simulink model "tqdtqr_rebuild_V3"  (R2021b)
settings: Solver=VariableStepAuto  StartTime=0.0  StopTime=10.0  RelTol=1e-3
undefined symbols (not defined in the file): ATQD_AfterTqMinGain_X_Deg, ATQD_APSCreepBaseTqD_X_kph, ATQD_APSCreepBaseTqD_Y_Deg, ATQD_APSCreepBaseTqR_X_kph, ATQD_APSCreepBaseTqR_Y_Deg, ATQD_APSCreepIterm_X_kph, ATQD_APSCreepIterm_Y_kph, ATQD_APSCreepPterm_X_kph, ATQD_APSCreepPterm_Y_kph, ATQD_APSDecReq_X_kph, ATQD_APSDecReq_Y_mps2, ATQD_APSDecReqCMD_X_kph, ATQD_APSDecReqTs_X_pct, ATQD_APSDecTimeGain_X_Deg, ATQD_APSDecTimeGain_Y_s, ATQD_APSReqLowSpd_X_Deg, ATQD_AutoHoldReleaseBPS_X_Deg, ATQD_AWDLoadTrqnsGain_X_kg, ATQD_AWDLoadTrqnsGain_Y_pct, ATQD_BOSEnBPSPosn_X_kph, ATQD_BOSMap_X_rpm, ATQD_BOSMap_Y_pct, ATQD_CreepBaseTqD_X_kph, ATQD_CreepBaseTqD_Y_Deg, ATQD_CreepBaseTqR_X_kph, ATQD_CreepBaseTqR_Y_Deg, ATQD_CreepBPSDisPosn_X_Deg, ATQD_CreepBPSDisPosnR_X_Deg, ATQD_CreepBPSEnPosn_X_Deg, ATQD_CreepBPSEnPosnR_X_Deg, ATQD_CreepDeltaTq_X_kph, ATQD_CreepIterm_X_kph, ATQD_CreepIterm_Y_kph, ATQD_CreepItermMaxLimit_X_pct, ATQD_CreepPreloadTime_X_kph, ATQD_CreepPreloadTq_X_kph, ATQD_CreepPreloadTq_Y_s, ATQD_CreepProtTq_X_Deg, ATQD_CreepPterm_X_kph, ATQD_CreepPterm_Y_kph, ATQD_CreepRrTqSpRat_X_rpm, ATQD_CreepRrTqSpRat_Y_Nm, ATQD_CreepTargetSpdD_X_pct, ATQD_CreepTargetSpdR_X_pct, ATQD_CreepUpLimitTq_X_rpm, ATQD_DecIneOPDHoldEnDelay_X_Deg, ATQD_DecIneOPDHoldEnDelay_Y_bar, ATQD_ECOTqMapD_X_rpm, ATQD_ECOTqMapD_Y_pct, ATQD_EMTqMapD_X_rpm, ATQD_EMTqMapD_Y_pct, ATQD_EOPDTqMapDCon_X_rpm, ATQD_EOPDTqMapDCon_Y_Deg, ATQD_EstInitVehWeight_X_c, ATQD_FAfterTqCMDGain_X_rpm, ATQD_FAfterTqCMDGain_Y_pct, ATQD_ForceLowSpd_X_Deg, ATQD_ForcePLimitSpd_X_Deg, ATQD_FrLossMAPLowV_X_rpm, ATQD_FrLossMAPLowV_Y_Nm ... (+949)
libraries: simulink x235, hcu_lib x208, tqr x63, tqd x6
(part 29 of 37)

== system tqdtqr_rebuild_V3/Input_Convert/Signal function/VehWeightEst/Calaulation/Rear Wheel Torque ==
  VINP_RrEDURealTMTq_Nm : Inport
  VTQD_VehWeightEstEn_flg : Inport  Port=2
  VTQD_VehWeightEstDis_flg : Inport  Port=3
  VTQD_VehWeightEstEnd_flg : Inport  Port=4
  task_time_s : Inport  Port=5
  AND : Logic  AllPortsSameDT=off  OutDataTypeStr=boolean
  AND1 : Logic  AllPortsSameDT=off  OutDataTypeStr=boolean
  AND2 : Logic  AllPortsSameDT=off  OutDataTypeStr=boolean
  Abs : Abs
  Add : Sum
  Add1 : Sum
  Add2 : Sum  Inputs=+-
  Constant1 : Constant  Value=ZERO_FLOAT
  Constant2 : Constant  Value=KTQD_VehWeighEstTime_s
  Constant3 : Constant  Value=ZERO_FLOAT
  Constant4 : Constant  Value=KTQD_VehWeighEstTimeTune_cnt
  Constant5 : Constant  Value=ZERO_FLOAT
  Constant6 : Constant  Value=KTQD_EstRrWhlTqDev_Nm
  Data Type Conversion : DataTypeConversion  OutDataTypeStr=uint8
  Delay : Delay  DelayLength=1  InitialCondition=boolean(0)
      settings: AttributesFormatString=%<InitialCondition>
  Delay1 : Delay  DelayLength=1  InitialCondition=single(0.0)
      settings: AttributesFormatString=%<InitialCondition>
  Delay2 : Delay  DelayLength=1
  Delay3 : Delay  DelayLength=1  InitialCondition=boolean(0)
      settings: AttributesFormatString=%<InitialCondition>
  Delay4 : Delay  DelayLength=1  InitialCondition=single(0.0)
      settings: AttributesFormatString=%<InitialCondition>
  Detect Decrease : simulink/Logic and Bit Operations/Detect Decrease  vinit=boolean(0)  OutDataTypeStr=boolean
  Detect Increase : simulink/Logic and Bit Operations/Detect Increase  vinit=boolean(0)  OutDataTypeStr=boolean
  Divide : Product  Inputs=*/
  Divide1 : Product  Inputs=*/
  Min : MinMax  Inputs=2
  NOT : Logic  Operator=NOT  AllPortsSameDT=off  OutDataTypeStr=boolean
  NOT1 : Logic  Operator=NOT  AllPortsSameDT=off  OutDataTypeStr=boolean
  Relational Operator : RelationalOperator  Operator=<=  OutDataTypeStr=boolean  RndMeth=Simplest
  Switch : Switch  Criteria=u2 ~= 0
  Switch1 : Switch  Criteria=u2 ~= 0
  Switch2 : Switch  Criteria=u2 > Threshold
  Switch3 : Switch  Criteria=u2 ~= 0
      settings: AttributesFormatString=%<Criteria>
  Terminator : Terminator
  VTQD_EstRrRealTqAvg_Nm : Outport
  VTQD_EstRrRealTqCheckPass_flg : Outport  Port=2
  wires:
  [VTQD_EstRrRealTqAvg_Nm] -> VTQD_EstRrRealTqAvg_Nm/1
  [VTQD_EstRrRealTqCheckPass_flg] -> VTQD_EstRrRealTqCheckPass_flg/1
  Constant4/1 -> Add1/2
  [VINP_RrEDURealTMTq_Nm] -> Min/1
  Delay1/1 -> Add/2
  Constant3/1 -> Switch2/1
  [VTQD_VehWeightEstEn_flg] -> AND/1
  Divide1/1 -> [VTQD_EstRrRealTqAvg_Nm]  "VTQD_EstRrRealTqAvg_Nm"
  Switch/1 -> Add/1
  [VTQD_EstRrRealTqSum_Nm] -> Divide1/1
  [VTQD_VehWeightEstEn_flg] -> Detect Decrease/1
  AND/1 -> Switch/2
  Constant1/1 -> Switch/3
  [VTQD_VehWeightEstEn_flg] -> Detect Increase/1
  Relational Operator/1 -> AND1/2
  Add/1 -> Switch1/3
  Constant6/1 -> Relational Operator/2
  [VTQD_EstRrRealTqAvg_Nm] -> Add2/1
  [VINP_RrEDURealTMTq_Nm] -> Switch/1
  NOT/1 -> AND/2
  Constant5/1 -> Switch1/1
  Switch1/1 -> [VTQD_EstRrRealTqSum_Nm], Delay1/1  "VTQD_EstRrRealTqSum_Nm"
  Switch2/1 -> Delay4/1, [VTQD_EstRrRealTqMin_Nm]  "VTQD_EstRrRealTqMin_Nm"
  Constant2/1 -> Divide/1
  [VTQD_EstRrRealTqMin_Nm] -> Add2/2
  [VTQD_VehWeightEstDis_flg] -> Delay/1
  Delay2/1 -> Min/2
  [VTQD_EstRrRealTqMin_Nm] -> Delay2/1
  [task_time_s] -> Divide/2
  Detect Increase/1 -> Switch2/2
  Delay/1 -> NOT/1
  Abs/1 -> Relational Operator/1
  Add2/1 -> Abs/1
  [VTQD_VehWeightEstDis_flg] -> AND1/1
  AND1/1 -> [VTQD_EstRrRealTqCheckPass_flg]  "VTQD_EstRrRealTqCheckPass_flg"
  VINP_RrEDURealTMTq_Nm/1 -> [VINP_RrEDURealTMTq_Nm]
  VTQD_VehWeightEstEn_flg/1 -> [VTQD_VehWeightEstEn_flg]
  VTQD_VehWeightEstDis_flg/1 -> [VTQD_VehWeightEstDis_flg]
  VTQD_VehWeightEstEnd_flg/1 -> Terminator/1
  task_time_s/1 -> [task_time_s]
  Add1/1 -> Divide1/2  "VTQD_EstCycleCount_cnt"
  Divide/1 -> Data Type Conversion/1
  Data Type Conversion/1 -> Add1/1
  [VTQD_VehWeightEstEn_flg] -> AND2/1
  NOT1/1 -> AND2/2
  Delay3/1 -> NOT1/1
  [VTQD_VehWeightEstDis_flg] -> Delay3/1
  AND2/1 -> Switch3/2
  Min/1 -> Switch3/1
  Switch3/1 -> Switch2/3
  Delay4/1 -> Switch3/3
  Detect Decrease/1 -> Switch1/2

== system tqdtqr_rebuild_V3/Input_Convert/Signal function/VehWeightEst/Calaulation/Vehicle Weight ==
  VTQD_EstFrRealTqAvg_Nm : Inport
  VTQD_EstRrRealTqAvg_Nm : Inport  Port=2
  VTQD_EstLongAccAvg_Gps : Inport  Port=3
  VINP_VehSpeed_kph : Inport  Port=4
  Add : Sum  Inputs=+++
  Add1 : Sum
  Add2 : Sum
  Add3 : Sum
  Constant1 : Constant  Value=KTQD_RrTMTotalGearRatio_gain
  Constant10 : Constant  Value=KTQR_FrTMGearEff_c
  Constant11 : Constant  Value=KTQR_RrTMGearEff_c
  Constant12 : Constant  Value=MINUSONE_FLOAT
  Constant13 : Constant  Value=KTQD_GravityValue_mps2
  Constant2 : Constant  Value=KTQD_FrTMTotalGearRatio_gain
  Constant3 : Constant  Value=MINUSONE_FLOAT
  Constant4 : Constant  Value=MINUSONE_FLOAT
  Constant5 : Constant  Value=KTQD_FrTireRadius_m
  Constant6 : Constant  Value=KTQD_RrTireRadius_m
  Constant7 : Constant  Value=KTQD_EstRollCoeffA_c
  Constant8 : Constant  Value=KTQD_EstRollCoeffB_c
  Constant9 : Constant  Value=KTQD_EstRollCoeffC_c
  Divide : Product  Inputs=*/
  Divide1 : Product  Inputs=*/
  Divide2 : Product  Inputs=*/
  Product{,3..5} (4 alike) : Product
  Product1 : Product  Inputs=3
  Product2 : Product  Inputs=3
  Product6 : Product  Inputs=3
  Square : Math  Operator=square  SaturateOnIntegerOverflow=on
  VTQD_EstVehWeight_kg : Outport
  wires:
  [VINP_VehSpeed_kph] -> Square/1
  Divide/1 -> Add1/1  "VTQD_EstFrForce_N"
  Product2/1 -> Divide2/1  "VTQD_EstRrWhlTqAvg_Nm"
  [VINP_VehSpeed_kph] -> Product/2
  Constant6/1 -> Divide2/2
  Product1/1 -> Divide/1  "VTQD_EstFrWhlTqAvg_Nm"
  Constant2/1 -> Product1/2
  Constant1/1 -> Product2/2
  Add1/1 -> Product4/1
  Square/1 -> Product3/2
  [VTQD_EstRrRealTqAvg_Nm] -> Product2/1
  Constant3/1 -> Product1/3
  [VTQD_EstRollForce_N] -> Add2/2
  Constant9/1 -> Product3/1
  Constant7/1 -> Add/1
  [VTQD_EstFrRealTqAvg_Nm] -> Product1/1
  Constant10/1 -> Product4/2
  Add2/1 -> Product5/1
  Product4/1 -> Add3/1  "VTQD_EstFrActForce_N"
  Constant5/1 -> Divide/2
  Add/1 -> [VTQD_EstRollForce_N]  "VTQD_EstRollForce_N"
  Product/1 -> Add/2
  Constant4/1 -> Product2/3
  Add3/1 -> [VTQD_EstActTotalForce_N]  "VTQD_EstActTotalForce_N"
  Product5/1 -> Add3/2  "VTQD_EstRrActForce_N"
  Constant8/1 -> Product/1
  Divide2/1 -> Add2/1  "VTQD_EstRrForce_N"
  Constant11/1 -> Product5/2
  [VTQD_EstRollForce_N] -> Add1/2
  Product3/1 -> Add/3
  [VTQD_EstLongAccAvg_Gps] -> Product6/1
  Constant12/1 -> Product6/2
  Product6/1 -> Divide1/2
  [VTQD_EstActTotalForce_N] -> Divide1/1
  VTQD_EstFrRealTqAvg_Nm/1 -> [VTQD_EstFrRealTqAvg_Nm]
  VTQD_EstRrRealTqAvg_Nm/1 -> [VTQD_EstRrRealTqAvg_Nm]
  VTQD_EstLongAccAvg_Gps/1 -> [VTQD_EstLongAccAvg_Gps]
  VINP_VehSpeed_kph/1 -> [VINP_VehSpeed_kph]
  [VTQD_EstVehWeight_kg] -> VTQD_EstVehWeight_kg/1
  Constant13/1 -> Product6/3
  Divide1/1 -> [VTQD_EstVehWeight_kg]  "VTQD_EstVehWeight_kg"

== system tqdtqr_rebuild_V3/Input_Convert/Signal function/combo key/Combo Key Detection/DiagnosisOff Mode ==
  note: Check value key1~8 and diagnosis off mode on
  note: Detect combo key value from key1~8
  note: Exhibition Mode:
      | 1 = VINP_SWC2RegenDown_flg
      | 2 = VINP_SWC2RegenUp_flg
      | 3 = VINP_SWC2LScrollUpSta_flg
      | 4 = VINP_SWC2LScrollDownSta_flg
      | 5 = VINP_SWC2RScrollUpSta_flg
      | 6 = VINP_SWC2RScrollDownSta_flg
      | 7 = VINP_SWC2LScrollPressSta_flg
      | 8 = VINP_SWC2LADASSta_flg
  TASK_TIME_10_MS : Inport
  VSCP_ComboKeyEn_flg : Inport  Port=2
  VSCP_ComboKeyReset_flg : Inport  Port=3
  VSCP_ComboKey_enum : Inport  Port=4
  VSCP_ComboKeyEnter_flg : Inport  Port=5
  VSCP_StreetFightModeOff_flg : Inport  Port=6
  AND : Logic  Inputs=9  AllPortsSameDT=off  OutDataTypeStr=boolean
  Constant : Constant  Value=ENUM_COMBOKEY_NONE
  Constant1 : Constant  Value=ENUM_COMBOKEY_NONE
  Constant2 : Constant  Value=FALSE
  Constant3 : Constant  Value=KTQD_ComboKeyDelay_s
  Delay : Delay  DelayLength=1  InitialCondition=boolean(0)
      settings: AttributesFormatString=%<InitialCondition>
  DelayEnable : hcu_lib/Basic_Blocks/DelayEnable
  Equal : RelationalOperator  Operator=~=  OutDataTypeStr=boolean  RndMeth=Simplest
  Key1 : Subsystem
  Key2 : Subsystem
  Key3 : Subsystem
  Key4 : Subsystem
  Key5 : Subsystem
  Key6 : Subsystem
  Key7 : Subsystem
  Key8 : Subsystem
  Switch : Switch  Criteria=u2 ~= 0
      settings: AttributesFormatString=%<Criteria>
  Switch1 : Switch  Criteria=u2 ~= 0
      settings: AttributesFormatString=%<Criteria>
  Switch2 : Switch  Criteria=u2 ~= 0
      settings: AttributesFormatString=%<Criteria>
  VSCP_DiagnosisOffMode_flg : Outport
  wires:
  [VSCP_DiagnosisOffMode_flg] -> VSCP_DiagnosisOffMode_flg/1
  Switch/1 -> [VSCP_ComboKeyCMD_enum]  "VTQD_DiagnosisOffCMD_enum"
  [TASK_TIME_10_MS] -> DelayEnable/3
  Constant/1 -> Switch/3
  DelayEnable/1 -> Switch/2
  [VSCP_ComboKeyEn_flg] -> DelayEnable/1
  Constant3/1 -> DelayEnable/2
  [VSCP_ComboKey_enum] -> Switch/1
  [VSCP_ComboKeyCMD_enum] -> Key1/1(VSCP_ComboKeyCMD_enum)
  [VSCP_ComboKeyEn_flg] -> Key1/2(VSCP_ComboKeyEn_flg)
  [VSCP_ComboKeyReset_flg] -> Key1/3(VSCP_ComboKeyReset_flg)
  [VSCP_ComboKeyCMD_enum] -> Key2/1(VSCP_ComboKeyCMD_enum)
  [VSCP_ComboKeyEn_flg] -> Key2/2(VSCP_ComboKeyEn_flg)
  [VSCP_ComboKeyReset_flg] -> Key2/3(VSCP_ComboKeyReset_flg)
  [VSCP_ComboKey1_enum] -> Key2/4(VSCP_ComboKey1_enum)
  Key1/1(VSCP_ComboKey1_enum) -> [VSCP_ComboKey1_enum]
  Key1/2(VSCP_Key1Pass_flg) -> [VSCP_Key1Pass_flg]
  [VSCP_ComboKeyCMD_enum] -> Key3/1(VSCP_ComboKeyCMD_enum)
  [VSCP_ComboKeyEn_flg] -> Key3/2(VSCP_ComboKeyEn_flg)
  [VSCP_ComboKeyReset_flg] -> Key3/3(VSCP_ComboKeyReset_flg)
  [VSCP_ComboKey2_enum] -> Key3/4(VSCP_ComboKey2_enum)
  [VSCP_ComboKeyCMD_enum] -> Key4/1(VSCP_ComboKeyCMD_enum)
  [VSCP_ComboKeyEn_flg] -> Key4/2(VSCP_ComboKeyEn_flg)
  [VSCP_ComboKeyReset_flg] -> Key4/3(VSCP_ComboKeyReset_flg)
  Key2/1(VSCP_ComboKey2_enum) -> [VSCP_ComboKey2_enum]
  Key2/2(VSCP_Key2Pass_flg) -> [VSCP_Key2Pass_flg]
  [VSCP_ComboKey3_enum] -> Key4/4(VSCP_ComboKey3_enum)
  Key3/1(VSCP_ComboKey3_enum) -> [VSCP_ComboKey3_enum]
  Key3/2(VSCP_Key3Pass_flg) -> [VSCP_Key3Pass_flg]
  Key4/1(VSCP_ComboKey4_enum) -> [VSCP_ComboKey4_enum]
  Key4/2(VSCP_Key4Pass_flg) -> [VSCP_Key4Pass_flg]
  [VSCP_ComboKeyReset_flg] -> Key5/3(VSCP_ComboKeyReset_flg)
  [VSCP_ComboKeyEn_flg] -> Key5/2(VSCP_ComboKeyEn_flg)
  [VSCP_ComboKeyCMD_enum] -> Key5/1(VSCP_ComboKeyCMD_enum)
  [VSCP_ComboKey4_enum] -> Key5/4(VSCP_ComboKey4_enum)
  Key5/2(VSCP_Key5Pass_flg) -> [VSCP_Key5Pass_flg]
  Key5/1(VSCP_ComboKey5_enum) -> [VSCP_ComboKey5_enum]
  Key7/2(VSCP_Key7Pass_flg) -> [VSCP_Key7Pass_flg]
  Key8/1(VSCP_ComboKey8_enum) -> [VSCP_ComboKey8_enum]
  Key8/2(VSCP_Key8Pass_flg) -> [VSCP_Key8Pass_flg]
  [VSCP_ComboKeyCMD_enum] -> Key6/1(VSCP_ComboKeyCMD_enum)
  [VSCP_ComboKeyEn_flg] -> Key6/2(VSCP_ComboKeyEn_flg)
  [VSCP_ComboKeyReset_flg] -> Key6/3(VSCP_ComboKeyReset_flg)
  [VSCP_ComboKey5_enum] -> Key6/4(VSCP_ComboKey5_enum)
  [VSCP_ComboKeyCMD_enum] -> Key7/1(VSCP_ComboKeyCMD_enum)
  [VSCP_ComboKeyEn_flg] -> Key7/2(VSCP_ComboKeyEn_flg)
  [VSCP_ComboKeyReset_flg] -> Key7/3(VSCP_ComboKeyReset_flg)
  [VSCP_ComboKey6_enum] -> Key7/4(VSCP_ComboKey6_enum)
  [VSCP_ComboKeyCMD_enum] -> Key8/1(VSCP_ComboKeyCMD_enum)
  [VSCP_ComboKeyEn_flg] -> Key8/2(VSCP_ComboKeyEn_flg)
  [VSCP_ComboKeyReset_flg] -> Key8/3(VSCP_ComboKeyReset_flg)
  [VSCP_ComboKey7_enum] -> Key8/4(VSCP_ComboKey7_enum)
  Constant1/1 -> Equal/2
  Equal/1 -> AND/1
  [VSCP_Key1Pass_flg] -> AND/2
  [VSCP_Key8Pass_flg] -> AND/9
  [VSCP_Key7Pass_flg] -> AND/8
  [VSCP_Key6Pass_flg] -> AND/7
  [VSCP_Key5Pass_flg] -> AND/6
  [VSCP_Key4Pass_flg] -> AND/5
  [VSCP_Key3Pass_flg] -> AND/4
  [VSCP_Key2Pass_flg] -> AND/3
  [VSCP_ComboKeyEnter_flg] -> Switch1/2
  AND/1 -> Switch1/1  "VTQD_DiagnosisOffPass_flg"
  Switch1/1 -> Switch2/3
  [VSCP_StreetFightModeOff_flg] -> Switch2/2
  Constant2/1 -> Switch2/1
  Switch2/1 -> Delay/1, [VSCP_DiagnosisOffMode_flg]  "VTQD_DiagnosisOffMode_flg"
  Delay/1 -> Switch1/3
  TASK_TIME_10_MS/1 -> [TASK_TIME_10_MS]
  VSCP_ComboKeyEn_flg/1 -> [VSCP_ComboKeyEn_flg]
  VSCP_ComboKeyReset_flg/1 -> [VSCP_ComboKeyReset_flg]
  VSCP_ComboKey_enum/1 -> [VSCP_ComboKey_enum]
  VSCP_ComboKeyEnter_flg/1 -> [VSCP_ComboKeyEnter_flg]
  VSCP_StreetFightModeOff_flg/1 -> [VSCP_StreetFightModeOff_flg]
  Key6/1(VSCP_ComboKey6_enum) -> [VSCP_ComboKey6_enum]
  Key6/2(VSCP_Key6Pass_flg) -> [VSCP_Key6Pass_flg]
  Key7/1(VSCP_ComboKey7_enum) -> [VSCP_ComboKey7_enum]
  [VSCP_ComboKey8_enum] -> Equal/1

== system tqdtqr_rebuild_V3/Input_Convert/Signal function/combo key/Combo Key Detection/Engineering Mode ==
  note: Check value key1~8 and engineering mode on
  note: Detect combo key value from key1~8
  note: Engineering Mode:
      | 5 = VINP_SWC2RScrollUpSta_flg
      | 5 = VINP_SWC2RScrollUpSta_flg
      | 6 = VINP_SWC2RScrollDownSta_flg
      | 6 = VINP_SWC2RScrollDownSta_flg
      | 5 = VINP_SWC2RScrollUpSta_flg
      | 6 = VINP_SWC2RScrollDownSta_flg
      | 5 = VINP_SWC2RScrollUpSta_flg
      | 6 = VINP_SWC2RScrollDownSta_flg
  TASK_TIME_10_MS : Inport
  VSCP_ComboKeyEn_flg : Inport  Port=2
  VSCP_ComboKeyReset_flg : Inport  Port=3
  VSCP_ComboKey_enum : Inport  Port=4
  VSCP_ComboKeyEnter_flg : Inport  Port=5
  VSCP_StreetFightModeOff_flg : Inport  Port=6
  AND : Logic  Inputs=9  AllPortsSameDT=off  OutDataTypeStr=boolean
  Constant : Constant  Value=ENUM_COMBOKEY_NONE
  Constant1 : Constant  Value=ENUM_COMBOKEY_NONE
  Constant2 : Constant  Value=FALSE
  Constant3 : Constant  Value=KTQD_ComboKeyDelay_s
  Delay : Delay  DelayLength=1  InitialCondition=boolean(0)
      settings: AttributesFormatString=%<InitialCondition>
  DelayEnable : hcu_lib/Basic_Blocks/DelayEnable
  Equal : RelationalOperator  Operator=~=  OutDataTypeStr=boolean  RndMeth=Simplest
  Key1 : Subsystem
  Key2 : Subsystem
  Key3 : Subsystem
  Key4 : Subsystem
  Key5 : Subsystem
  Key6 : Subsystem
  Key7 : Subsystem
  Key8 : Subsystem
  Switch : Switch  Criteria=u2 ~= 0
      settings: AttributesFormatString=%<Criteria>
  Switch1 : Switch  Criteria=u2 ~= 0
      settings: AttributesFormatString=%<Criteria>
  Switch2 : Switch  Criteria=u2 ~= 0
      settings: AttributesFormatString=%<Criteria>
  VSCP_EngineeringMode_flg : Outport
  wires:
  [VSCP_ComboKey8_enum] -> Equal/1
  Key7/1(VSCP_ComboKey7_enum) -> [VSCP_ComboKey7_enum]
  Key6/2(VSCP_Key6Pass_flg) -> [VSCP_Key6Pass_flg]
  Key6/1(VSCP_ComboKey6_enum) -> [VSCP_ComboKey6_enum]
  VSCP_StreetFightModeOff_flg/1 -> [VSCP_StreetFightModeOff_flg]
  VSCP_ComboKeyEnter_flg/1 -> [VSCP_ComboKeyEnter_flg]
  VSCP_ComboKey_enum/1 -> [VSCP_ComboKey_enum]
  VSCP_ComboKeyReset_flg/1 -> [VSCP_ComboKeyReset_flg]
  VSCP_ComboKeyEn_flg/1 -> [VSCP_ComboKeyEn_flg]
  TASK_TIME_10_MS/1 -> [TASK_TIME_10_MS]
  Delay/1 -> Switch1/3
  Switch2/1 -> [VSCP_EngineeringMode_flg], Delay/1  "VTQD_EngineeringMode_flg"
  Constant2/1 -> Switch2/1
  [VSCP_StreetFightModeOff_flg] -> Switch2/2
  Switch1/1 -> Switch2/3
  AND/1 -> Switch1/1  "VTQD_EngineeringPass_flg"
  [VSCP_ComboKeyEnter_flg] -> Switch1/2
  [VSCP_Key2Pass_flg] -> AND/3
  [VSCP_Key3Pass_flg] -> AND/4
  [VSCP_Key4Pass_flg] -> AND/5
  [VSCP_Key5Pass_flg] -> AND/6
  [VSCP_Key6Pass_flg] -> AND/7
  [VSCP_Key7Pass_flg] -> AND/8
  [VSCP_Key8Pass_flg] -> AND/9
  [VSCP_Key1Pass_flg] -> AND/2
  Equal/1 -> AND/1
  Constant1/1 -> Equal/2
  [VSCP_ComboKey7_enum] -> Key8/4(VSCP_ComboKey7_enum)
  [VSCP_ComboKeyReset_flg] -> Key8/3(VSCP_ComboKeyReset_flg)
  [VSCP_ComboKeyEn_flg] -> Key8/2(VSCP_ComboKeyEn_flg)
  [VSCP_ComboKeyCMD_enum] -> Key8/1(VSCP_ComboKeyCMD_enum)
  [VSCP_ComboKey6_enum] -> Key7/4(VSCP_ComboKey6_enum)
  [VSCP_ComboKeyReset_flg] -> Key7/3(VSCP_ComboKeyReset_flg)
  [VSCP_ComboKeyEn_flg] -> Key7/2(VSCP_ComboKeyEn_flg)
  [VSCP_ComboKeyCMD_enum] -> Key7/1(VSCP_ComboKeyCMD_enum)
  [VSCP_ComboKey5_enum] -> Key6/4(VSCP_ComboKey5_enum)
  [VSCP_ComboKeyReset_flg] -> Key6/3(VSCP_ComboKeyReset_flg)
  [VSCP_ComboKeyEn_flg] -> Key6/2(VSCP_ComboKeyEn_flg)
  [VSCP_ComboKeyCMD_enum] -> Key6/1(VSCP_ComboKeyCMD_enum)
  Key8/2(VSCP_Key8Pass_flg) -> [VSCP_Key8Pass_flg]
  Key8/1(VSCP_ComboKey8_enum) -> [VSCP_ComboKey8_enum]
  Key7/2(VSCP_Key7Pass_flg) -> [VSCP_Key7Pass_flg]
  Key5/1(VSCP_ComboKey5_enum) -> [VSCP_ComboKey5_enum]
  Key5/2(VSCP_Key5Pass_flg) -> [VSCP_Key5Pass_flg]
  [VSCP_ComboKey4_enum] -> Key5/4(VSCP_ComboKey4_enum)
  [VSCP_ComboKeyCMD_enum] -> Key5/1(VSCP_ComboKeyCMD_enum)
  [VSCP_ComboKeyEn_flg] -> Key5/2(VSCP_ComboKeyEn_flg)
  [VSCP_ComboKeyReset_flg] -> Key5/3(VSCP_ComboKeyReset_flg)
  Key4/2(VSCP_Key4Pass_flg) -> [VSCP_Key4Pass_flg]
  Key4/1(VSCP_ComboKey4_enum) -> [VSCP_ComboKey4_enum]
  Key3/2(VSCP_Key3Pass_flg) -> [VSCP_Key3Pass_flg]
  Key3/1(VSCP_ComboKey3_enum) -> [VSCP_ComboKey3_enum]
  [VSCP_ComboKey3_enum] -> Key4/4(VSCP_ComboKey3_enum)
  Key2/2(VSCP_Key2Pass_flg) -> [VSCP_Key2Pass_flg]
  Key2/1(VSCP_ComboKey2_enum) -> [VSCP_ComboKey2_enum]
  [VSCP_ComboKeyReset_flg] -> Key4/3(VSCP_ComboKeyReset_flg)
  [VSCP_ComboKeyEn_flg] -> Key4/2(VSCP_ComboKeyEn_flg)
  [VSCP_ComboKeyCMD_enum] -> Key4/1(VSCP_ComboKeyCMD_enum)
  [VSCP_ComboKey2_enum] -> Key3/4(VSCP_ComboKey2_enum)
  [VSCP_ComboKeyReset_flg] -> Key3/3(VSCP_ComboKeyReset_flg)
  [VSCP_ComboKeyEn_flg] -> Key3/2(VSCP_ComboKeyEn_flg)
  [VSCP_ComboKeyCMD_enum] -> Key3/1(VSCP_ComboKeyCMD_enum)
  Key1/2(VSCP_Key1Pass_flg) -> [VSCP_Key1Pass_flg]
  Key1/1(VSCP_ComboKey1_enum) -> [VSCP_ComboKey1_enum]
  [VSCP_ComboKey1_enum] -> Key2/4(VSCP_ComboKey1_enum)
  [VSCP_ComboKeyReset_flg] -> Key2/3(VSCP_ComboKeyReset_flg)
  [VSCP_ComboKeyEn_flg] -> Key2/2(VSCP_ComboKeyEn_flg)
  [VSCP_ComboKeyCMD_enum] -> Key2/1(VSCP_ComboKeyCMD_enum)
  [VSCP_ComboKeyReset_flg] -> Key1/3(VSCP_ComboKeyReset_flg)
  [VSCP_ComboKeyEn_flg] -> Key1/2(VSCP_ComboKeyEn_flg)
  [VSCP_ComboKeyCMD_enum] -> Key1/1(VSCP_ComboKeyCMD_enum)
  [VSCP_ComboKey_enum] -> Switch/1
  Constant3/1 -> DelayEnable/2
  [VSCP_ComboKeyEn_flg] -> DelayEnable/1
  DelayEnable/1 -> Switch/2
  Constant/1 -> Switch/3
  [TASK_TIME_10_MS] -> DelayEnable/3
  Switch/1 -> [VSCP_ComboKeyCMD_enum]  "VTQD_EngineeringCMD_enum"
  [VSCP_EngineeringMode_flg] -> VSCP_EngineeringMode_flg/1

== system tqdtqr_rebuild_V3/Input_Convert/Signal function/combo key/Combo Key Detection/Exhibition Mode ==
  note: Check value key1~8 and exhibition mode on
  note: Detect combo key value from key1~8
  note: Exhibition Mode:
      | 7 = VINP_SWC2LScrollPressSta_flg
      | 7 = VINP_SWC2LScrollPressSta_flg
      | 8 = VINP_SWC2LADASSta_flg
      | 8 = VINP_SWC2LADASSta_flg
      | 8 = VINP_SWC2LADASSta_flg
      | 7 = VINP_SWC2LScrollPressSta_flg
      | 8 = VINP_SWC2LADASSta_flg
      | 7 = VINP_SWC2LScrollPressSta_flg
  TASK_TIME_10_MS : Inport
  VSCP_ComboKeyEn_flg : Inport  Port=2
  VSCP_ComboKeyReset_flg : Inport  Port=3
  VSCP_ComboKey_enum : Inport  Port=4
  VSCP_ComboKeyEnter_flg : Inport  Port=5
  VSCP_StreetFightModeOff_flg : Inport  Port=6
  AND : Logic  Inputs=9  AllPortsSameDT=off  OutDataTypeStr=boolean
  Constant : Constant  Value=ENUM_COMBOKEY_NONE
  Constant1 : Constant  Value=ENUM_COMBOKEY_NONE
  Constant2 : Constant  Value=FALSE
  Constant3 : Constant  Value=KTQD_ComboKeyDelay_s
  Delay : Delay  DelayLength=1  InitialCondition=boolean(0)
      settings: AttributesFormatString=%<InitialCondition>
  DelayEnable : hcu_lib/Basic_Blocks/DelayEnable
  Equal : RelationalOperator  Operator=~=  OutDataTypeStr=boolean  RndMeth=Simplest
  Key1 : Subsystem
  Key2 : Subsystem
  Key3 : Subsystem
  Key4 : Subsystem
  Key5 : Subsystem
  Key6 : Subsystem
  Key7 : Subsystem
  Key8 : Subsystem
  Switch : Switch  Criteria=u2 ~= 0
      settings: AttributesFormatString=%<Criteria>
  Switch1 : Switch  Criteria=u2 ~= 0
      settings: AttributesFormatString=%<Criteria>
  Switch2 : Switch  Criteria=u2 ~= 0
      settings: AttributesFormatString=%<Criteria>
  VSCP_ExhibitionMode_flg : Outport
  wires:
  [VSCP_ComboKey8_enum] -> Equal/1
  Key7/1(VSCP_ComboKey7_enum) -> [VSCP_ComboKey7_enum]
  Key6/2(VSCP_Key6Pass_flg) -> [VSCP_Key6Pass_flg]
  Key6/1(VSCP_ComboKey6_enum) -> [VSCP_ComboKey6_enum]
  VSCP_StreetFightModeOff_flg/1 -> [VSCP_StreetFightModeOff_flg]
  VSCP_ComboKeyEnter_flg/1 -> [VSCP_ComboKeyEnter_flg]
  VSCP_ComboKey_enum/1 -> [VSCP_ComboKey_enum]
  VSCP_ComboKeyReset_flg/1 -> [VSCP_ComboKeyReset_flg]
  VSCP_ComboKeyEn_flg/1 -> [VSCP_ComboKeyEn_flg]
  TASK_TIME_10_MS/1 -> [TASK_TIME_10_MS]
  Delay/1 -> Switch1/3
  Switch2/1 -> [VSCP_ExhibitionMode_flg], Delay/1  "VTQD_ExhibitionMode_flg"
  Constant2/1 -> Switch2/1
  [VSCP_StreetFightModeOff_flg] -> Switch2/2
  Switch1/1 -> Switch2/3
  AND/1 -> Switch1/1  "VTQD_ExhibitionPass_flg"
  [VSCP_ComboKeyEnter_flg] -> Switch1/2
  [VSCP_Key2Pass_flg] -> AND/3
  [VSCP_Key3Pass_flg] -> AND/4
  [VSCP_Key4Pass_flg] -> AND/5
  [VSCP_Key5Pass_flg] -> AND/6
  [VSCP_Key6Pass_flg] -> AND/7
  [VSCP_Key7Pass_flg] -> AND/8
  [VSCP_Key8Pass_flg] -> AND/9
  [VSCP_Key1Pass_flg] -> AND/2
  Equal/1 -> AND/1
  Constant1/1 -> Equal/2
  [VSCP_ComboKey7_enum] -> Key8/4(VSCP_ComboKey7_enum)
  [VSCP_ComboKeyReset_flg] -> Key8/3(VSCP_ComboKeyReset_flg)
  [VSCP_ComboKeyEn_flg] -> Key8/2(VSCP_ComboKeyEn_flg)
  [VSCP_ComboKeyCMD_enum] -> Key8/1(VSCP_ComboKeyCMD_enum)
  [VSCP_ComboKey6_enum] -> Key7/4(VSCP_ComboKey6_enum)
  [VSCP_ComboKeyReset_flg] -> Key7/3(VSCP_ComboKeyReset_flg)
  [VSCP_ComboKeyEn_flg] -> Key7/2(VSCP_ComboKeyEn_flg)
  [VSCP_ComboKeyCMD_enum] -> Key7/1(VSCP_ComboKeyCMD_enum)
  [VSCP_ComboKey5_enum] -> Key6/4(VSCP_ComboKey5_enum)
  [VSCP_ComboKeyReset_flg] -> Key6/3(VSCP_ComboKeyReset_flg)
  [VSCP_ComboKeyEn_flg] -> Key6/2(VSCP_ComboKeyEn_flg)
  [VSCP_ComboKeyCMD_enum] -> Key6/1(VSCP_ComboKeyCMD_enum)
  Key8/2(VSCP_Key8Pass_flg) -> [VSCP_Key8Pass_flg]
  Key8/1(VSCP_ComboKey8_enum) -> [VSCP_ComboKey8_enum]
  Key7/2(VSCP_Key7Pass_flg) -> [VSCP_Key7Pass_flg]
  Key5/1(VSCP_ComboKey5_enum) -> [VSCP_ComboKey5_enum]
  Key5/2(VSCP_Key5Pass_flg) -> [VSCP_Key5Pass_flg]
  [VSCP_ComboKey4_enum] -> Key5/4(VSCP_ComboKey4_enum)
  [VSCP_ComboKeyCMD_enum] -> Key5/1(VSCP_ComboKeyCMD_enum)
  [VSCP_ComboKeyEn_flg] -> Key5/2(VSCP_ComboKeyEn_flg)
  [VSCP_ComboKeyReset_flg] -> Key5/3(VSCP_ComboKeyReset_flg)
  Key4/2(VSCP_Key4Pass_flg) -> [VSCP_Key4Pass_flg]
  Key4/1(VSCP_ComboKey4_enum) -> [VSCP_ComboKey4_enum]
  Key3/2(VSCP_Key3Pass_flg) -> [VSCP_Key3Pass_flg]
  Key3/1(VSCP_ComboKey3_enum) -> [VSCP_ComboKey3_enum]
  [VSCP_ComboKey3_enum] -> Key4/4(VSCP_ComboKey3_enum)
  Key2/2(VSCP_Key2Pass_flg) -> [VSCP_Key2Pass_flg]
  Key2/1(VSCP_ComboKey2_enum) -> [VSCP_ComboKey2_enum]
  [VSCP_ComboKeyReset_flg] -> Key4/3(VSCP_ComboKeyReset_flg)
  [VSCP_ComboKeyEn_flg] -> Key4/2(VSCP_ComboKeyEn_flg)
  [VSCP_ComboKeyCMD_enum] -> Key4/1(VSCP_ComboKeyCMD_enum)
  [VSCP_ComboKey2_enum] -> Key3/4(VSCP_ComboKey2_enum)
  [VSCP_ComboKeyReset_flg] -> Key3/3(VSCP_ComboKeyReset_flg)
  [VSCP_ComboKeyEn_flg] -> Key3/2(VSCP_ComboKeyEn_flg)
  [VSCP_ComboKeyCMD_enum] -> Key3/1(VSCP_ComboKeyCMD_enum)
  Key1/2(VSCP_Key1Pass_flg) -> [VSCP_Key1Pass_flg]
  Key1/1(VSCP_ComboKey1_enum) -> [VSCP_ComboKey1_enum]
  [VSCP_ComboKey1_enum] -> Key2/4(VSCP_ComboKey1_enum)
  [VSCP_ComboKeyReset_flg] -> Key2/3(VSCP_ComboKeyReset_flg)
  [VSCP_ComboKeyEn_flg] -> Key2/2(VSCP_ComboKeyEn_flg)
  [VSCP_ComboKeyCMD_enum] -> Key2/1(VSCP_ComboKeyCMD_enum)
  [VSCP_ComboKeyReset_flg] -> Key1/3(VSCP_ComboKeyReset_flg)
  [VSCP_ComboKeyEn_flg] -> Key1/2(VSCP_ComboKeyEn_flg)
  [VSCP_ComboKeyCMD_enum] -> Key1/1(VSCP_ComboKeyCMD_enum)
  [VSCP_ComboKey_enum] -> Switch/1
  Constant3/1 -> DelayEnable/2
  [VSCP_ComboKeyEn_flg] -> DelayEnable/1
  DelayEnable/1 -> Switch/2
  Constant/1 -> Switch/3
  [TASK_TIME_10_MS] -> DelayEnable/3
  Switch/1 -> [VSCP_ComboKeyCMD_enum]  "VTQD_ExhibitionCMD_enum"
  [VSCP_ExhibitionMode_flg] -> VSCP_ExhibitionMode_flg/1

== system tqdtqr_rebuild_V3/Input_Convert/Signal function/combo key/Combo Key Detection/Manufacture Mode ==
  note: Check value key1~8 and manufacture mode on
  note: Detect combo key value from key1~8
  note: Manufacture Mode:
      | 11 = VINP_SWC2RRightSta_flg
      | 12 = VINP_SWC2RLeftSta_flg
      | 11 = VINP_SWC2RRightSta_flg
      | 12 = VINP_SWC2RLeftSta_flg
      | 11 = VINP_SWC2RRightSta_flg
      | 12 = VINP_SWC2RLeftSta_flg
      | 7 = VINP_SWC2LScrollPressSta_flg
      | 8 = VINP_SWC2LADASSta_flg
  TASK_TIME_10_MS : Inport
  VSCP_ComboKeyEn_flg : Inport  Port=2
  VSCP_ComboKeyReset_flg : Inport  Port=3
  VSCP_ComboKey_enum : Inport  Port=4
  VSCP_ComboKeyEnter_flg : Inport  Port=5
  VSCP_StreetFightModeOff_flg : Inport  Port=6
  AND : Logic  Inputs=9  AllPortsSameDT=off  OutDataTypeStr=boolean
  Constant : Constant  Value=ENUM_COMBOKEY_NONE
  Constant1 : Constant  Value=ENUM_COMBOKEY_NONE
  Constant2 : Constant  Value=FALSE
  Constant3 : Constant  Value=KTQD_ComboKeyDelay_s
  Delay : Delay  DelayLength=1  InitialCondition=boolean(0)
      settings: AttributesFormatString=%<InitialCondition>
  DelayEnable : hcu_lib/Basic_Blocks/DelayEnable
  Equal : RelationalOperator  Operator=~=  OutDataTypeStr=boolean  RndMeth=Simplest
  Key1 : Subsystem
  Key2 : Subsystem
  Key3 : Subsystem
  Key4 : Subsystem
  Key5 : Subsystem
  Key6 : Subsystem
  Key7 : Subsystem
  Key8 : Subsystem
  Switch : Switch  Criteria=u2 ~= 0
      settings: AttributesFormatString=%<Criteria>
  Switch1 : Switch  Criteria=u2 ~= 0
      settings: AttributesFormatString=%<Criteria>
  Switch2 : Switch  Criteria=u2 ~= 0
      settings: AttributesFormatString=%<Criteria>
  VSCP_ManufactureMode_flg : Outport
  wires:
  [VSCP_ManufactureMode_flg] -> VSCP_ManufactureMode_flg/1
  Switch/1 -> [VSCP_ComboKeyCMD_enum]  "VTQD_ManufactureCMD_enum"
  [TASK_TIME_10_MS] -> DelayEnable/3
  Constant/1 -> Switch/3
  DelayEnable/1 -> Switch/2
  [VSCP_ComboKeyEn_flg] -> DelayEnable/1
  Constant3/1 -> DelayEnable/2
  [VSCP_ComboKey_enum] -> Switch/1
  [VSCP_ComboKeyCMD_enum] -> Key1/1(VSCP_ComboKeyCMD_enum)
  [VSCP_ComboKeyEn_flg] -> Key1/2(VSCP_ComboKeyEn_flg)
  [VSCP_ComboKeyReset_flg] -> Key1/3(VSCP_ComboKeyReset_flg)
  [VSCP_ComboKeyCMD_enum] -> Key2/1(VSCP_ComboKeyCMD_enum)
  [VSCP_ComboKeyEn_flg] -> Key2/2(VSCP_ComboKeyEn_flg)
  [VSCP_ComboKeyReset_flg] -> Key2/3(VSCP_ComboKeyReset_flg)
  [VSCP_ComboKey1_enum] -> Key2/4(VSCP_ComboKey1_enum)
  Key1/1(VSCP_ComboKey1_enum) -> [VSCP_ComboKey1_enum]
  Key1/2(VSCP_Key1Pass_flg) -> [VSCP_Key1Pass_flg]
  [VSCP_ComboKeyCMD_enum] -> Key3/1(VSCP_ComboKeyCMD_enum)
  [VSCP_ComboKeyEn_flg] -> Key3/2(VSCP_ComboKeyEn_flg)
  [VSCP_ComboKeyReset_flg] -> Key3/3(VSCP_ComboKeyReset_flg)
  [VSCP_ComboKey2_enum] -> Key3/4(VSCP_ComboKey2_enum)
  [VSCP_ComboKeyCMD_enum] -> Key4/1(VSCP_ComboKeyCMD_enum)
  [VSCP_ComboKeyEn_flg] -> Key4/2(VSCP_ComboKeyEn_flg)
  [VSCP_ComboKeyReset_flg] -> Key4/3(VSCP_ComboKeyReset_flg)
  Key2/1(VSCP_ComboKey2_enum) -> [VSCP_ComboKey2_enum]
  Key2/2(VSCP_Key2Pass_flg) -> [VSCP_Key2Pass_flg]
  [VSCP_ComboKey3_enum] -> Key4/4(VSCP_ComboKey3_enum)
  Key3/1(VSCP_ComboKey3_enum) -> [VSCP_ComboKey3_enum]
  Key3/2(VSCP_Key3Pass_flg) -> [VSCP_Key3Pass_flg]
  Key4/1(VSCP_ComboKey4_enum) -> [VSCP_ComboKey4_enum]
  Key4/2(VSCP_Key4Pass_flg) -> [VSCP_Key4Pass_flg]
  [VSCP_ComboKeyReset_flg] -> Key5/3(VSCP_ComboKeyReset_flg)
  [VSCP_ComboKeyEn_flg] -> Key5/2(VSCP_ComboKeyEn_flg)
  [VSCP_ComboKeyCMD_enum] -> Key5/1(VSCP_ComboKeyCMD_enum)
  [VSCP_ComboKey4_enum] -> Key5/4(VSCP_ComboKey4_enum)
  Key5/2(VSCP_Key5Pass_flg) -> [VSCP_Key5Pass_flg]
  Key5/1(VSCP_ComboKey5_enum) -> [VSCP_ComboKey5_enum]
  Key7/2(VSCP_Key7Pass_flg) -> [VSCP_Key7Pass_flg]
  Key8/1(VSCP_ComboKey8_enum) -> [VSCP_ComboKey8_enum]
  Key8/2(VSCP_Key8Pass_flg) -> [VSCP_Key8Pass_flg]
  [VSCP_ComboKeyCMD_enum] -> Key6/1(VSCP_ComboKeyCMD_enum)
  [VSCP_ComboKeyEn_flg] -> Key6/2(VSCP_ComboKeyEn_flg)
  [VSCP_ComboKeyReset_flg] -> Key6/3(VSCP_ComboKeyReset_flg)
  [VSCP_ComboKey5_enum] -> Key6/4(VSCP_ComboKey5_enum)
  [VSCP_ComboKeyCMD_enum] -> Key7/1(VSCP_ComboKeyCMD_enum)
  [VSCP_ComboKeyEn_flg] -> Key7/2(VSCP_ComboKeyEn_flg)
  [VSCP_ComboKeyReset_flg] -> Key7/3(VSCP_ComboKeyReset_flg)
  [VSCP_ComboKey6_enum] -> Key7/4(VSCP_ComboKey6_enum)
  [VSCP_ComboKeyCMD_enum] -> Key8/1(VSCP_ComboKeyCMD_enum)
  [VSCP_ComboKeyEn_flg] -> Key8/2(VSCP_ComboKeyEn_flg)
  [VSCP_ComboKeyReset_flg] -> Key8/3(VSCP_ComboKeyReset_flg)
  [VSCP_ComboKey7_enum] -> Key8/4(VSCP_ComboKey7_enum)
  Constant1/1 -> Equal/2
  Equal/1 -> AND/1
  [VSCP_Key1Pass_flg] -> AND/2
  [VSCP_Key8Pass_flg] -> AND/9
  [VSCP_Key7Pass_flg] -> AND/8
  [VSCP_Key6Pass_flg] -> AND/7
  [VSCP_Key5Pass_flg] -> AND/6
  [VSCP_Key4Pass_flg] -> AND/5
  [VSCP_Key3Pass_flg] -> AND/4
  [VSCP_Key2Pass_flg] -> AND/3
  [VSCP_ComboKeyEnter_flg] -> Switch1/2
  AND/1 -> Switch1/1  "VTQD_ManufacturePass_flg"
  Switch1/1 -> Switch2/3
  [VSCP_StreetFightModeOff_flg] -> Switch2/2
  Constant2/1 -> Switch2/1
  Switch2/1 -> Delay/1, [VSCP_ManufactureMode_flg]  "VTQD_ManufactureMode_flg"
  Delay/1 -> Switch1/3
  TASK_TIME_10_MS/1 -> [TASK_TIME_10_MS]
  VSCP_ComboKeyEn_flg/1 -> [VSCP_ComboKeyEn_flg]
  VSCP_ComboKeyReset_flg/1 -> [VSCP_ComboKeyReset_flg]
  VSCP_ComboKey_enum/1 -> [VSCP_ComboKey_enum]
  VSCP_ComboKeyEnter_flg/1 -> [VSCP_ComboKeyEnter_flg]
  VSCP_StreetFightModeOff_flg/1 -> [VSCP_StreetFightModeOff_flg]
  Key6/1(VSCP_ComboKey6_enum) -> [VSCP_ComboKey6_enum]
  Key6/2(VSCP_Key6Pass_flg) -> [VSCP_Key6Pass_flg]
  Key7/1(VSCP_ComboKey7_enum) -> [VSCP_ComboKey7_enum]
  [VSCP_ComboKey8_enum] -> Equal/1

== system tqdtqr_rebuild_V3/Input_Convert/Signal function/combo key/Combo Key Detection/Street Fight Mode ==
  note: Check value key1~8 and street fight mode on
  note: Detect combo key value from key1~8
  note: Street Fight Mode:
      | 3 = VINP_SWC2LScrollUpSta_flg
      | 3 = VINP_SWC2LScrollUpSta_flg
      | 4 = VINP_SWC2LScrollDownSta_flg
      | 4 = VINP_SWC2LScrollDownSta_flg
      | 1 = VINP_SWC2RegenDown_flg
      | 1 = VINP_SWC2RegenDown_flg
      | 2 = VINP_SWC2RegenUp_flg
      | 2 = VINP_SWC2RegenUp_flg
  TASK_TIME_10_MS : Inport
  VSCP_ComboKeyEn_flg : Inport  Port=2
  VSCP_ComboKeyReset_flg : Inport  Port=3
  VSCP_ComboKey_enum : Inport  Port=4
  VSCP_ComboKeyEnter_flg : Inport  Port=5
  VSCP_StreetFightModeOff_flg : Inport  Port=6
  AND : Logic  Inputs=9  AllPortsSameDT=off  OutDataTypeStr=boolean
  Constant : Constant  Value=ENUM_COMBOKEY_NONE
  Constant1 : Constant  Value=ENUM_COMBOKEY_NONE
  Constant2 : Constant  Value=FALSE
  Constant3 : Constant  Value=KTQD_ComboKeyDelay_s
  Delay : Delay  DelayLength=1  InitialCondition=boolean(0)
      settings: AttributesFormatString=%<InitialCondition>
  DelayEnable : hcu_lib/Basic_Blocks/DelayEnable
  Equal : RelationalOperator  Operator=~=  OutDataTypeStr=boolean  RndMeth=Simplest
  Key1 : Subsystem
  Key2 : Subsystem
  Key3 : Subsystem
  Key4 : Subsystem
  Key5 : Subsystem
  Key6 : Subsystem
  Key7 : Subsystem
  Key8 : Subsystem
  Switch : Switch  Criteria=u2 ~= 0
      settings: AttributesFormatString=%<Criteria>
  Switch1 : Switch  Criteria=u2 ~= 0
      settings: AttributesFormatString=%<Criteria>
  Switch2 : Switch  Criteria=u2 ~= 0
      settings: AttributesFormatString=%<Criteria>
  VSCP_StreetFightMode_flg : Outport
  wires:
  Switch/1 -> [VSCP_ComboKeyCMD_enum]  "VTQD_StreetFightCMD_enum"
  [TASK_TIME_10_MS] -> DelayEnable/3
  Constant/1 -> Switch/3
  DelayEnable/1 -> Switch/2
  [VSCP_ComboKeyEn_flg] -> DelayEnable/1
  Constant3/1 -> DelayEnable/2
  [VSCP_ComboKey_enum] -> Switch/1
  [VSCP_ComboKeyCMD_enum] -> Key1/1(VSCP_ComboKeyCMD_enum)
  [VSCP_ComboKeyEn_flg] -> Key1/2(VSCP_ComboKeyEn_flg)
  [VSCP_ComboKeyReset_flg] -> Key1/3(VSCP_ComboKeyReset_flg)
  [VSCP_ComboKeyCMD_enum] -> Key2/1(VSCP_ComboKeyCMD_enum)
  [VSCP_ComboKeyEn_flg] -> Key2/2(VSCP_ComboKeyEn_flg)
  [VSCP_ComboKeyReset_flg] -> Key2/3(VSCP_ComboKeyReset_flg)
  [VSCP_ComboKey1_enum] -> Key2/4(VSCP_ComboKey1_enum)
  Key1/1(VSCP_ComboKey1_enum) -> [VSCP_ComboKey1_enum]
  Key1/2(VSCP_Key1Pass_flg) -> [VSCP_Key1Pass_flg]
  [VSCP_ComboKeyCMD_enum] -> Key3/1(VSCP_ComboKeyCMD_enum)
  [VSCP_ComboKeyEn_flg] -> Key3/2(VSCP_ComboKeyEn_flg)
  [VSCP_ComboKeyReset_flg] -> Key3/3(VSCP_ComboKeyReset_flg)
  [VSCP_ComboKey2_enum] -> Key3/4(VSCP_ComboKey2_enum)
  [VSCP_ComboKeyCMD_enum] -> Key4/1(VSCP_ComboKeyCMD_enum)
  [VSCP_ComboKeyEn_flg] -> Key4/2(VSCP_ComboKeyEn_flg)
  [VSCP_ComboKeyReset_flg] -> Key4/3(VSCP_ComboKeyReset_flg)
  Key2/1(VSCP_ComboKey2_enum) -> [VSCP_ComboKey2_enum]
  Key2/2(VSCP_Key2Pass_flg) -> [VSCP_Key2Pass_flg]
  [VSCP_ComboKey3_enum] -> Key4/4(VSCP_ComboKey3_enum)
  Key3/1(VSCP_ComboKey3_enum) -> [VSCP_ComboKey3_enum]
  Key3/2(VSCP_Key3Pass_flg) -> [VSCP_Key3Pass_flg]
  Key4/1(VSCP_ComboKey4_enum) -> [VSCP_ComboKey4_enum]
  Key4/2(VSCP_Key4Pass_flg) -> [VSCP_Key4Pass_flg]
  [VSCP_ComboKeyReset_flg] -> Key5/3(VSCP_ComboKeyReset_flg)
  [VSCP_ComboKeyEn_flg] -> Key5/2(VSCP_ComboKeyEn_flg)
  [VSCP_ComboKeyCMD_enum] -> Key5/1(VSCP_ComboKeyCMD_enum)
  [VSCP_ComboKey4_enum] -> Key5/4(VSCP_ComboKey4_enum)
  Key5/2(VSCP_Key5Pass_flg) -> [VSCP_Key5Pass_flg]
  Key5/1(VSCP_ComboKey5_enum) -> [VSCP_ComboKey5_enum]
  Key7/2(VSCP_Key7Pass_flg) -> [VSCP_Key7Pass_flg]
  Key8/1(VSCP_ComboKey8_enum) -> [VSCP_ComboKey8_enum]
  Key8/2(VSCP_Key8Pass_flg) -> [VSCP_Key8Pass_flg]
  [VSCP_ComboKeyCMD_enum] -> Key6/1(VSCP_ComboKeyCMD_enum)
  [VSCP_ComboKeyEn_flg] -> Key6/2(VSCP_ComboKeyEn_flg)
  [VSCP_ComboKeyReset_flg] -> Key6/3(VSCP_ComboKeyReset_flg)
  [VSCP_ComboKey5_enum] -> Key6/4(VSCP_ComboKey5_enum)
  [VSCP_ComboKeyCMD_enum] -> Key7/1(VSCP_ComboKeyCMD_enum)
  [VSCP_ComboKeyEn_flg] -> Key7/2(VSCP_ComboKeyEn_flg)
  [VSCP_ComboKeyReset_flg] -> Key7/3(VSCP_ComboKeyReset_flg)
  [VSCP_ComboKey6_enum] -> Key7/4(VSCP_ComboKey6_enum)
  [VSCP_ComboKeyCMD_enum] -> Key8/1(VSCP_ComboKeyCMD_enum)
  [VSCP_ComboKeyEn_flg] -> Key8/2(VSCP_ComboKeyEn_flg)
  [VSCP_ComboKeyReset_flg] -> Key8/3(VSCP_ComboKeyReset_flg)
  [VSCP_ComboKey7_enum] -> Key8/4(VSCP_ComboKey7_enum)
  Constant1/1 -> Equal/2
  Equal/1 -> AND/1
  [VSCP_Key1Pass_flg] -> AND/2
  [VSCP_Key8Pass_flg] -> AND/9
  [VSCP_Key7Pass_flg] -> AND/8
  [VSCP_Key6Pass_flg] -> AND/7
  [VSCP_Key5Pass_flg] -> AND/6
  [VSCP_Key4Pass_flg] -> AND/5
  [VSCP_Key3Pass_flg] -> AND/4
  [VSCP_Key2Pass_flg] -> AND/3
  [VSCP_ComboKeyEnter_flg] -> Switch1/2
  AND/1 -> Switch1/1  "VTQD_StreetFightPass_flg"
  Switch1/1 -> Switch2/3
  [VSCP_StreetFightModeOff_flg] -> Switch2/2
  Constant2/1 -> Switch2/1
  Switch2/1 -> Delay/1, [VSCP_StreetFightMode_flg]  "VTQD_StreetFightMode_flg"
  Delay/1 -> Switch1/3
  TASK_TIME_10_MS/1 -> [TASK_TIME_10_MS]
  VSCP_ComboKeyEn_flg/1 -> [VSCP_ComboKeyEn_flg]
  VSCP_ComboKeyReset_flg/1 -> [VSCP_ComboKeyReset_flg]
  VSCP_ComboKey_enum/1 -> [VSCP_ComboKey_enum]
  VSCP_ComboKeyEnter_flg/1 -> [VSCP_ComboKeyEnter_flg]
  VSCP_StreetFightModeOff_flg/1 -> [VSCP_StreetFightModeOff_flg]
  [VSCP_StreetFightMode_flg] -> VSCP_StreetFightMode_flg/1
  Key6/1(VSCP_ComboKey6_enum) -> [VSCP_ComboKey6_enum]
  Key6/2(VSCP_Key6Pass_flg) -> [VSCP_Key6Pass_flg]
  Key7/1(VSCP_ComboKey7_enum) -> [VSCP_ComboKey7_enum]
  [VSCP_ComboKey8_enum] -> Equal/1

== system tqdtqr_rebuild_V3/Input_Convert/Signal function/combo key/Mode Coordination/DiagnosisOff ==
  Action Port : ActionPort  ActionPortLabel=elseif( u5 ~= 0)
  Constant : Constant  Value=ENUM_SYSMODE_DIAGNOSISOFF
  DiagnosisOff : Outport
  wires:
  Constant/1 -> DiagnosisOff/1

== system tqdtqr_rebuild_V3/Input_Convert/Signal function/combo key/Mode Coordination/Engineering ==
  Action Port : ActionPort  ActionPortLabel=elseif(u2 ~= 0)
  Constant : Constant  Value=ENUM_SYSMODE_ENGINEERING
  Engineering : Outport
  wires:
  Constant/1 -> Engineering/1

== system tqdtqr_rebuild_V3/Input_Convert/Signal function/combo key/Mode Coordination/Exhibition ==
  Action Port : ActionPort  ActionPortLabel=elseif( u4 ~= 0)
  Constant : Constant  Value=ENUM_SYSMODE_EXHIBITION
  Exhibition : Outport
  wires:
  Constant/1 -> Exhibition/1

== system tqdtqr_rebuild_V3/Input_Convert/Signal function/combo key/Mode Coordination/Manufacture ==
  Action Port : ActionPort  ActionPortLabel=elseif( u3 ~= 0)
  Constant : Constant  Value=ENUM_SYSMODE_MANUFACTURE
  Manufacture : Outport
  wires:
  Constant/1 -> Manufacture/1

== system tqdtqr_rebuild_V3/Input_Convert/Signal function/combo key/Mode Coordination/Product ==
  Action Port : ActionPort  ActionPortLabel=else
  Constant : Constant  Value=ENUM_SYSMODE_PRODUCT
  Product : Outport
  wires:
  Constant/1 -> Product/1

== system tqdtqr_rebuild_V3/Input_Convert/Signal function/combo key/Mode Coordination/StreetFight ==
  Action Port : ActionPort  ActionPortLabel=if(u1 ~=0)
  Constant : Constant  Value=ENUM_SYSMODE_DEVELOPING
  StreetFight : Outport
  wires:
  Constant/1 -> StreetFight/1

== system tqdtqr_rebuild_V3/Input_Convert/Signal function/combo key/Signal Status Detection/None ==
  Action Port : ActionPort  ActionPortLabel=else
  Constant : Constant  Value=ENUM_COMBOKEY_NONE  OutDataTypeStr=uint8
  None_enum : Outport
  wires:
  Constant/1 -> None_enum/1

== system tqdtqr_rebuild_V3/Input_Convert/Signal function/combo key/Signal Status Detection/SWCACCSta ==
  Action Port : ActionPort  ActionPortLabel=elseif(u8~=0)
  Constant : Constant  Value=ENUM_COMBOKEY_SWCACC  OutDataTypeStr=uint8
  SWCACCSta_enum : Outport
  wires:
  Constant/1 -> SWCACCSta_enum/1

== system tqdtqr_rebuild_V3/Input_Convert/Signal function/combo key/Signal Status Detection/SWCCANCELStaShort ==
  Action Port : ActionPort  ActionPortLabel=elseif(u7 ~=0)
  Constant : Constant  Value=ENUM_COMBOKEY_CANCEL  OutDataTypeStr=uint8
  SWCCANCELStaShort_enum : Outport
  wires:
  Constant/1 -> SWCCANCELStaShort_enum/1

== system tqdtqr_rebuild_V3/Input_Convert/Signal function/combo key/Signal Status Detection/SWCDistanceSta ==
  Action Port : ActionPort  ActionPortLabel=elseif(u9~=0)
  Constant : Constant  Value=ENUM_COMBOKEY_DISTANCE  OutDataTypeStr=uint8
  SWCDownStaShort_enum : Outport
  wires:
  Constant/1 -> SWCDownStaShort_enum/1

== system tqdtqr_rebuild_V3/Input_Convert/Signal function/combo key/Signal Status Detection/SWCDownStaShort ==
  Action Port : ActionPort  ActionPortLabel=elseif(u6~=0)
  Constant : Constant  Value=ENUM_COMBOKEY_SWCDOWN  OutDataTypeStr=uint8
  SWCDownStaShort_enum : Outport
  wires:
  Constant/1 -> SWCDownStaShort_enum/1

== system tqdtqr_rebuild_V3/Input_Convert/Signal function/combo key/Signal Status Detection/SWCLeftSta ==
  Action Port : ActionPort  ActionPortLabel=elseif(u12~=0)
  Constant : Constant  Value=ENUM_COMBOKEY_SWCLEFT  OutDataTypeStr=uint8
  SWCLeftSta_enum : Outport
  wires:
  Constant/1 -> SWCLeftSta_enum/1

== system tqdtqr_rebuild_V3/Input_Convert/Signal function/combo key/Signal Status Detection/SWCRegenDownShort ==
  Action Port : ActionPort  ActionPortLabel=if(u1~=0)
  Constant : Constant  Value=ENUM_COMBOKEY_REGENDOWN  OutDataTypeStr=uint8
  SWCRegenDownShort_enum : Outport
  wires:
  Constant/1 -> SWCRegenDownShort_enum/1

== system tqdtqr_rebuild_V3/Input_Convert/Signal function/combo key/Signal Status Detection/SWCRegenUpShort ==
  Action Port : ActionPort  ActionPortLabel=elseif(u2~=0)
  Constant : Constant  Value=ENUM_COMBOKEY_REGENUP  OutDataTypeStr=uint8
  SWCRegenUpShort_enum : Outport
  wires:
  Constant/1 -> SWCRegenUpShort_enum/1

== system tqdtqr_rebuild_V3/Input_Convert/Signal function/combo key/Signal Status Detection/SWCResUpStaShort ==
  Action Port : ActionPort  ActionPortLabel=elseif(u3~=0)
  Constant : Constant  Value=ENUM_COMBOKEY_RESUP  OutDataTypeStr=uint8
  SWCResUpStaShort_enum : Outport
  wires:
  Constant/1 -> SWCResUpStaShort_enum/1

== system tqdtqr_rebuild_V3/Input_Convert/Signal function/combo key/Signal Status Detection/SWCRightSta ==
  Action Port : ActionPort  ActionPortLabel=elseif(u11~=0)
  Constant : Constant  Value=ENUM_COMBOKEY_SWCRIGHT  OutDataTypeStr=uint8
  SWCRightSta_enum : Outport
  wires:
  Constant/1 -> SWCRightSta_enum/1

== system tqdtqr_rebuild_V3/Input_Convert/Signal function/combo key/Signal Status Detection/SWCSetdownStaShort ==
  Action Port : ActionPort  ActionPortLabel=elseif(u4~=0)
  Constant : Constant  Value=ENUM_COMBOKEY_SETDOWN  OutDataTypeStr=uint8
  SWCSetdownStaShort_enum : Outport
  wires:
  Constant/1 -> SWCSetdownStaShort_enum/1

== system tqdtqr_rebuild_V3/Input_Convert/Signal function/combo key/Signal Status Detection/SWCUpStaShort ==
  Action Port : ActionPort  ActionPortLabel=elseif(u5~=0)
  Constant : Constant  Value=ENUM_COMBOKEY_SWCUP  OutDataTypeStr=uint8
  SWCUpStaShort_enum : Outport
  wires:
  Constant/1 -> SWCUpStaShort_enum/1

== system tqdtqr_rebuild_V3/Input_Convert/Signal function/combo key/Signal Status Detection/SWCmodeSta ==
  Action Port : ActionPort  ActionPortLabel=elseif(u10~=0)
  Constant : Constant  Value=ENUM_COMBOKEY_SWCMODE  OutDataTypeStr=uint8
  SWCmodeSta_enum : Outport
  wires:
  Constant/1 -> SWCmodeSta_enum/1

== system tqdtqr_rebuild_V3/Input_Convert/Signal function/combo key/Signal Status Detection/Street Fight Switch Off ==
  TASK_TIME_10_MS : Inport
  VSCP_SWCCANCELStaShort_flg : Inport  Port=2
  VSCP_ComboKeyPreEn_flg : Inport  Port=3
  SWCCANCELStaLong_flg : Inport  Port=4
  VSCP_SysMode_enum : Inport  Port=5
  AND : Logic  AllPortsSameDT=off  OutDataTypeStr=boolean
  AND2 : Logic  AllPortsSameDT=off  OutDataTypeStr=boolean
  Add : Sum
  Constant1 : Constant  Value=ZERO_INT
  Constant11 : Constant  Value=ONE_INT
  Constant2 : Constant  Value=ONE_INT
  Constant3 : Constant  Value=KTQD_CANCELUpCount_cnt
  Constant4 : Constant  Value=ZERO_INT
  Constant5 : Constant  Value=ENUM_SYSMODE_PRODUCT
  Constant7 : Constant  Value=KTQD_CANCELCountDetTime_s
  Delay : Delay  DelayLength=1  InitialCondition=uint8(0)
      settings: AttributesFormatString=%<InitialCondition>
  Delay1 : Delay  DelayLength=1  InitialCondition=boolean(0)
      settings: AttributesFormatString=%<InitialCondition>
  Delay2 : Delay  DelayLength=1
  Delay3 : Delay  DelayLength=1  InitialCondition=uint8(0)
      settings: AttributesFormatString=%<InitialCondition>
  Equal : RelationalOperator  Operator===  OutDataTypeStr=boolean  RndMeth=Simplest
  Equal1 : RelationalOperator  Operator===  OutDataTypeStr=boolean  RndMeth=Simplest
  Equal2 : RelationalOperator  Operator===  OutDataTypeStr=boolean  RndMeth=Simplest
  NOT : Logic  Operator=NOT  AllPortsSameDT=off  OutDataTypeStr=boolean
  NOT1 : Logic  Operator=NOT  AllPortsSameDT=off  OutDataTypeStr=boolean
  OR : Logic  Operator=OR  Inputs=3  AllPortsSameDT=off  OutDataTypeStr=boolean
  Relational Operator : RelationalOperator  OutDataTypeStr=boolean  RndMeth=Simplest
  SR_Latch : hcu_lib/Basic_Blocks/SR_Latch
  Switch : Switch  Criteria=u2 ~= 0
      settings: AttributesFormatString=%<Criteria>
  Switch1 : Switch  Criteria=u2 ~= 0
      settings: AttributesFormatString=%<Criteria>
  Timer : hcu_lib/Basic_Blocks/Timer
  VSCP_StreetFightModeOff_flg : Outport
  wires:
  Constant1/1 -> Switch/3
  [VSCP_SWCCANCELStaShort_flg] -> Switch/2
  Constant11/1 -> Switch/1
  Switch/1 -> Add/1
  Add/1 -> Switch1/3
  Switch1/1 -> [VSCP_CANCELCount_cnt], Delay/1  "VTQD_CANCELCount_cnt"
  Delay/1 -> Add/2
  [VSCP_CANCELCount_cnt] -> Equal/1
  Constant2/1 -> Equal/2
  Equal/1 -> AND/1
  [VSCP_ComboKeyPreEn_flg] -> AND/2
  AND/1 -> SR_Latch/1
  SR_Latch/1 -> NOT/1, Timer/1
  NOT/1 -> Timer/2
  [TASK_TIME_10_MS] -> Timer/3
  Constant7/1 -> Relational Operator/2, Timer/4
  Timer/1 -> Relational Operator/1  "VTQD_CANCELCountDetTime_s"
  Relational Operator/1 -> [VSCP_CANCELCountDetFinish_flg]  "VTQD_CANCELCountDetFinish_flg"
  [VSCP_CANCELCount_cnt] -> Equal1/1
  Constant3/1 -> Equal1/2
  [SWCCANCELStaLong_flg] -> AND2/2
  [VSCP_CANCELCountDetFinish_flg] -> Delay1/1
  Delay1/1 -> SR_Latch/2
  [VSCP_CANCELCountDetFinish_flg] -> Delay2/1
  Constant4/1 -> Switch1/1
  Equal1/1 -> AND2/1
  AND2/1 -> [VSCP_StreetFightModeOff_flg]  "VTQD_StreetFightModeOff_flg"
  TASK_TIME_10_MS/1 -> [TASK_TIME_10_MS]
  VSCP_SWCCANCELStaShort_flg/1 -> [VSCP_SWCCANCELStaShort_flg]
  VSCP_ComboKeyPreEn_flg/1 -> [VSCP_ComboKeyPreEn_flg]
  SWCCANCELStaLong_flg/1 -> [SWCCANCELStaLong_flg]
  [VSCP_StreetFightModeOff_flg] -> VSCP_StreetFightModeOff_flg/1
  [VSCP_ComboKeyPreEn_flg] -> NOT1/1
  VSCP_SysMode_enum/1 -> [VSCP_SysMode_enum]
  Equal2/1 -> OR/1
  NOT1/1 -> OR/2
  Delay2/1 -> OR/3
  OR/1 -> [VSCP_CANCELCountReset_flg]  "VTQD_CANCELCountReset_flg"
  [VSCP_CANCELCountReset_flg] -> Switch1/2
  [VSCP_SysMode_enum] -> Delay3/1
  Delay3/1 -> Equal2/2
  Constant5/1 -> Equal2/1

== system tqdtqr_rebuild_V3/Input_Convert/Main function/DriverWhlTqDem function/Driver mode determination/NoLHM ShiftR/If Action Subsystem ==
  In1 : Inport
  Inport : Inport  Port=2
  Action Port : ActionPort  ActionPortLabel="if(u1 ~=  0)"
  MTQD_NRMOPDTqMapR_Z_Nm : Lookup_n-D  BreakpointsForDimension1=ATQD_NL1TqMapD_Y_pct  BreakpointsForDimension2=ATQD_NL1TqMapD_X_rpm  Table=MTQD_NRMOPDTqMapR_Z_Nm  ExtrapMethod=Clip  InternalRulePriority=Speed  RndMeth=Simplest  InputSameDT=on
      settings: InputPortMap=u0,u1
  Out1 : Outport
  wires:
  In1/1 -> MTQD_NRMOPDTqMapR_Z_Nm/1
  Inport/1 -> MTQD_NRMOPDTqMapR_Z_Nm/2
  MTQD_NRMOPDTqMapR_Z_Nm/1 -> Out1/1

== system tqdtqr_rebuild_V3/Input_Convert/Main function/DriverWhlTqDem function/Driver mode determination/NoLHM ShiftR/If Action Subsystem1 ==
  In1 : Inport
  Inport : Inport  Port=2
  Action Port : ActionPort  ActionPortLabel=else
  MTQD_NRMTqMapR_Z_Nm : Lookup_n-D  BreakpointsForDimension1=ATQD_NL1TqMapD_Y_pct  BreakpointsForDimension2=ATQD_NL1TqMapD_X_rpm  Table=MTQD_NRMTqMapR_Z_Nm  ExtrapMethod=Clip  InternalRulePriority=Speed  RndMeth=Simplest  InputSameDT=on
      settings: InputPortMap=u0,u1
  Out1 : Outport
  wires:
  In1/1 -> MTQD_NRMTqMapR_Z_Nm/1
  Inport/1 -> MTQD_NRMTqMapR_Z_Nm/2
  MTQD_NRMTqMapR_Z_Nm/1 -> Out1/1
